simulink model "Converter_Buck_with_signals"  (R2018a)
settings: Solver=ode23tb  StartTime=0.0  StopTime=0.01  MaxStep=10e-6  RelTol=1e-3
libraries: powerlib x13, simulink x1
settings Model: Creator=bw_  LastModifiedBy=bw_
settings SolverCC: InitialStep=10e-8

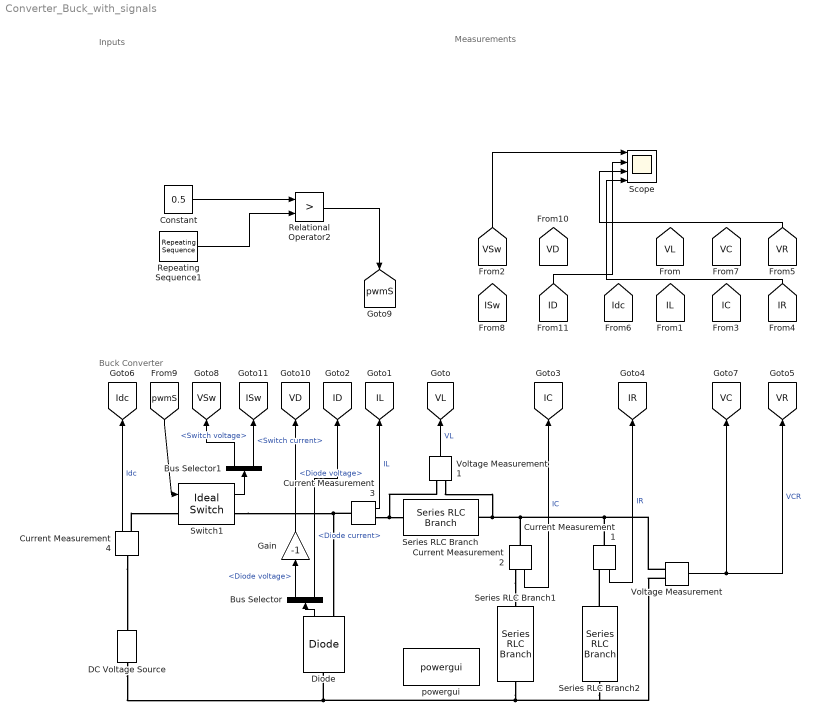
== system Converter_Buck_with_signals ==
  note: Inputs
  note: Measurements
  note: Buck Converter
  Bus Selector : BusSelector  OutputSignals=Diode voltage,Diode current
  Bus Selector1 : BusSelector  OutputSignals=Switch voltage,Switch current
  Constant : Constant  Value=0.5
  Current Measurement{1..4} (4 alike) : powerlib/Measurements/Current Measurement  PhasorSimulation=off  OutputType=Complex  PSBequivalent=0
  DC Voltage Source : powerlib/Electrical Sources/DC Voltage Source  Amplitude=100  Measurements=None
  Diode : powerlib/Power Electronics/Diode  Ron=0.001  Lon=0  Vf=0.8  IC=0  UseSnubber=0  Rs=500  Cs=250e-9  Measurements=on
  Gain : Gain  Gain=-1
  Relational Operator2 : RelationalOperator  Operator=>  OutDataTypeStr=boolean  RndMeth=Simplest
  Repeating Sequence1 : simulink/Sources/Repeating Sequence  rep_seq_t=[0 1/4 3/4 1]*(1/1000)  rep_seq_y=[1/2 1 0 1/2]
  Scope : Scope  NumInputPorts=4
  Series RLC Branch : powerlib/Elements/Series RLC Branch  LConnTagsString=__new0  RConnTagsString=__new0  BranchType=L  Resistance=1  Inductance=1e-3  SetiL0=off  InitialCurrent=0  Capacitance=1e-6  Setx0=off  InitialVoltage=0  Measurements=None
  Series RLC Branch1 : powerlib/Elements/Series RLC Branch  LConnTagsString=__new0  RConnTagsString=__new0  BranchType=C  Resistance=1  Inductance=1e-3  SetiL0=off  InitialCurrent=0  Capacitance=1e-6  Setx0=off  InitialVoltage=0  Measurements=None
  Series RLC Branch2 : powerlib/Elements/Series RLC Branch  LConnTagsString=__new0  RConnTagsString=__new0  BranchType=R  Resistance=50  Inductance=1e-3  SetiL0=off  InitialCurrent=0  Capacitance=1e-6  Setx0=off  InitialVoltage=0  Measurements=None
  Switch1 : powerlib/Power Electronics/Ideal Switch  Ron=0.001  Lon=0  IC=0  Rs=1e5  Cs=inf  Measurements=on
  Voltage Measurement : powerlib/Measurements/Voltage Measurement  PhasorSimulation=off  OutputType=Complex  PSBequivalent=0
  Voltage Measurement1 : powerlib/Measurements/Voltage Measurement  PhasorSimulation=off  OutputType=Complex  PSBequivalent=0
  powergui : powerlib/powergui  Priority=1  SimulationMode=Continuous  SampleTime=50e-6  frequency=60  Iterations=50  frequencyindice=0  Pbase=100e6  ErrMax=1e-4  UnitsV=kV  UnitsW=MW  buscounter=0  FunctionMessages=off  echomessages=off  EnableUseOfTLC=off  CurrentSourceSwitches=off  DisableSnubberDevices=off  DisableRonSwitches=off  DisableVfSwitches=off  DisplayEquations=off  SolverType=Tustin/Backward Euler (TBE)  Interpol=off  ExternalGateDelay=off  methode=off  Ts=100  x0status=blocks  SPID=on  SwTol=0  HookPort=off  RestoreLinks=warning  ResistiveCurrentMeasurement=off  Frange=[0:2:500]  Ylog=off  Xlog=on  ShowGrid=off  save=off  variable=ZData  structure=0  ZoomFFT=off  StartTime=0.0  cycles=1  DisplayStyle=1  fundamental=60  FreqAxis=off  MaxFrequency=1000  frequencyindicesteady=1  RmsSteady=1  display=off
  tag scope: IC=global, ID=global, IL=global, IR=global, ISw=global, Idc=global, VC=global, VD=global, VL=global, VR=global, VSw=global, pwmS=global
  wires:
  Current Measurement2/1 -> [IC]  "IC"
  Switch1/1 -> Bus Selector1/1
  Voltage Measurement/1 -> [VR], [VC]  "VCR"
  [pwmS] -> Switch1/1
  Current Measurement1/1 -> [IR]  "IR"
  Current Measurement4/1 -> [Idc]  "Idc"
  Current Measurement3/1 -> [IL]  "IL"
  Diode/1 -> Bus Selector/1
  Voltage Measurement1/1 -> [VL]  "VL"
  Bus Selector/2 -> [ID]  "<Diode current>"
  Bus Selector/1 -> Gain/1  "<Diode voltage>"
  Bus Selector1/2 -> [ISw]  "<Switch current>"
  Bus Selector1/1 -> [VSw]  "<Switch voltage>"
  Relational Operator2/1 -> [pwmS]
  Constant/1 -> Relational Operator2/1
  Repeating Sequence1/1 -> Relational Operator2/2
  [VSw] -> Scope/1
  [VR] -> Scope/3
  [ID] -> Scope/2
  Gain/1 -> [VD]  "<Diode voltage>"
  [IR] -> Scope/4
  connections:
  Series RLC Branch2/LConn1 -- Current Measurement1/RConn1
  Current Measurement3/RConn1 -- Voltage Measurement1/LConn1 -- Series RLC Branch/LConn1
  Current Measurement4/LConn1 -- DC Voltage Source/RConn1
  Voltage Measurement/LConn1 -- Current Measurement1/LConn1 -- Current Measurement2/LConn1 -- Voltage Measurement1/LConn2 -- Series RLC Branch/RConn1
  Current Measurement2/RConn1 -- Series RLC Branch1/LConn1
  DC Voltage Source/LConn1 -- Voltage Measurement/LConn2 -- Series RLC Branch2/RConn1 -- Series RLC Branch1/RConn1 -- Diode/LConn1
  Current Measurement4/RConn1 -- Switch1/LConn1
  Switch1/RConn1 -- Current Measurement3/LConn1 -- Diode/RConn1
